simulink model "PubIfDecisionLSM_MDL"  (R2020b)
settings: configuration reference "DspaceConfig" (kept outside this file)
PostLoadFcn:
  | if any(exist('dsrtsu_mdlpostloadfcn', 'file') ~= 0), dsrtsu_mdlpostloadfcn('Execute', bdroot); end
InitFcn:
  | , if any(exist('rtifpga_mdlclblib', 'file') ~= 0), rtifpga_mdlclblib('Init', bdroot); end,
  | , if any(exist('dsmpb_private', 'file') ~= 0), dsmpb_private('dsmpb_mdlclblib', 'Init', bdroot); end,
values from neighbouring files (symbols this model uses):
  P_LSM_ALC_Enable = 0.0    [LSM_Parameter.sldd]
  P_LSM_AwayEdge_offset = 0.1    [LSM_Parameter.sldd]
  P_LSM_CentValidErr = 1.0    [LSM_Parameter.sldd]
  P_LSM_DOP_C0_EN_Limit = 0.8    [LSM_Parameter.sldd]
  P_LSM_DOP_C0_out_Limit = 2.0    [LSM_Parameter.sldd]
  P_LSM_DOP_C1_EN_Limit : value not decoded    [LSM_Parameter.sldd]
  P_LSM_DOP_C1_out_Limit : value not decoded    [LSM_Parameter.sldd]
  P_LSM_DOP_C1AndC2_Lim_X : value not decoded    [LSM_Parameter.sldd]
  P_LSM_DOP_C2_EN_Limit : value not decoded    [LSM_Parameter.sldd]
  P_LSM_DOP_C2_out_Limit : value not decoded    [LSM_Parameter.sldd]
  P_LSM_DOP_In_Pre2Dop_Dis = 1.0    [LSM_Parameter.sldd]
  P_LSM_DOP_Out_Pre2Dop_Dis = 2.0    [LSM_Parameter.sldd]
  P_LSM_DOP_PreDis_X : value not decoded    [LSM_Parameter.sldd]
  P_LSM_DOP_PreDis_Y : value not decoded    [LSM_Parameter.sldd]
  P_LSM_DOPEnableSW = 1.0    [LSM_Parameter.sldd]
  P_LSM_DOPValid_CheckTime = 0.06    [LSM_Parameter.sldd]
  P_LSM_DoubleLine_Curr2Cent_Dislimit = 0.5    [LSM_Parameter.sldd]
  P_LSM_DoubleLine_Dop2Cent_Dislimit = 0.5    [LSM_Parameter.sldd]
  P_LSM_DoubleLine_DOPOut_C1 : value not decoded    [LSM_Parameter.sldd]
  P_LSM_DoubleLine_Pre2Cent_Dislimit = 1.0    [LSM_Parameter.sldd]
  P_LSM_Error_Limit = 0.5    [LSM_Parameter.sldd]
  P_LSM_IFV2CenterAxis = 0.0    [LSM_Parameter.sldd]
  P_LSM_IFV2RearAxis = 0.0    [LSM_Parameter.sldd]
  P_LSM_Line2Edge_limit = 0.5    [LSM_Parameter.sldd]
  P_LSM_Line_Error = 0.1    [LSM_Parameter.sldd]
  P_LSM_LineSTD_Limit = 0.15    [LSM_Parameter.sldd]
  P_LSM_NOH_Switch = 0.0    [LSM_Parameter.sldd]
  P_LSM_OTL_C0_Factor = 1.0    [LSM_Parameter.sldd]
  P_LSM_OTL_C1_Factor = 0.5    [LSM_Parameter.sldd]
  P_LSM_OTL_C2_Factor = 0.5    [LSM_Parameter.sldd]
  P_LSM_Pre2OnlyLineDis = 5.0    [LSM_Parameter.sldd]
  P_LSM_Pre_t = 0.0    [LSM_Parameter.sldd]
  P_LSM_SingleLine_Cent2Edge_Dislimit = 100.0    [LSM_Parameter.sldd]
  P_LSM_SingleLine_Curr2Cent_Dislimit = 0.2    [LSM_Parameter.sldd]
  P_LSM_SingleLine_Dop2Cent_Dislimit = 0.2    [LSM_Parameter.sldd]
  P_LSM_SingleLine_DOPOut_C1 : value not decoded    [LSM_Parameter.sldd]
  P_LSM_SingleLine_Pre2Cent_Dislimit = 0.5    [LSM_Parameter.sldd]
  P_LSM_TJALimitSpd = 60.0    [LSM_Parameter.sldd]
undefined symbols (not defined in the file or in its folder): P_lCS_IFV2CenterAxis, P_LCS_IFV2RearAxis, P_LSM_EntryEdge_offset, P_LSM_EntryLnChngEnSwitch, P_LSM_EntryVanishDis, P_LSM_LinetLostTime, P_LSM_LineWijCal_C12, P_LSM_LineWijCal_C13, P_LSM_MapValid_ErrorSwitch, P_LSM_PosLineLcFac, P_LSM_SpdLim_Stub_Spd, P_LSM_SpdLim_StubLength, P_LSM_SpdTurnAlarm
libraries: simulink x324, TrueDurationTime x11
(part 17 of 25)

== matlab function PubIfDecisionLSM_MDL/Subsystem1/TargetLineCalc_20ms2/LHLine ==
  data: LH_Count input; LH1A0 input single size=1; LH1A1 input single size=1; LH1A2 input single size=1; LH1A3 input single size=1; LH1RaMin input single size=1; LH1RaMax input single size=1; LH1Conf output uint8 size=1; LH1Avail input uint8 size=1; LH1LineType input uint8 size=1; LH1DLType input uint8 size=1; LH1SideType input uint8 size=1; LH1Wid input single size=1; LH1Crossing input; LH1Confidence input; LH1_Color input; LH1DEType input; LH2A0 input single size=1; LH2A1 input single size=1; LH2A2 input single size=1; LH2A3 input single size=1; LH2RaMin input single size=1; LH2RaMax input single size=1; LH2Avail input uint8 size=1; LH2LineType input uint8 size=1; LH2DLType input uint8 size=1; LH2SideType input uint8 size=1; LH2Wid input single size=1; LH1C0 output single size=1; LH1C1 output single size=1; LH1C2 output single size=1; LH1C3 output single size=1; LH1DxMin output single size=1; LH1DxMax output single size=1; LH1Type output uint8 size=1; LH1DLM output uint8 size=1; LH1Width output single size=1; LH1Reliable output; LeftLaneChange output uint8 size=1; LH1Color output; LH1DECEL output; LH2Conf output uint8 size=1; LH2C0 output single size=1; LH2C1 output single size=1; LH2C2 output single size=1; LH2C3 output single size=1; LH2DxMin output single size=1; LH2DxMax output single size=1; LH2Type output uint8 size=1; LH2DLM output uint8 size=1; LH2Width output single size=1; LH2Reliable output; RightLaneChange output uint8 size=1; LH2Crossing input; LH2Confidence input; LH2_Color input; LH2Color output; LH2DEType input; LH2DECEL output
function [LH1Conf,LH1C0,LH1C1,LH1C2,LH1C3,LH1DxMin,LH1DxMax,LH1Type,LH1DLM,LH1Width,LH1Reliable,LeftLaneChange,LH1Color,LH1DECEL,...
    LH2Conf,LH2C0,LH2C1,LH2C2,LH2C3,LH2DxMin,LH2DxMax,LH2Type,LH2DLM,LH2Width,LH2Reliable,RightLaneChange,LH2Color,LH2DECEL]...
    = LH(LH_Count,LH1A0,LH1A1,LH1A2,LH1A3,LH1RaMin,LH1RaMax,LH1Avail,LH1LineType,LH1DLType,LH1SideType,LH1Wid,LH1Crossing,LH1Confidence,LH1_Color,LH1DEType,...
    LH2A0,LH2A1,LH2A2,LH2A3,LH2RaMin,LH2RaMax,LH2Avail,LH2LineType,LH2DLType,LH2SideType,LH2Wid,LH2Crossing,LH2Confidence,LH2_Color,LH2DEType)

LH1Conf = uint8(0);
LH1C0 = single(0);
LH1C1 = single(0);
LH1C2 = single(0);
LH1C3 = single(0);
LH1DxMin = single(0);
LH1DxMax = single(0);
LH1Type = uint8(0);
LH1DLM = uint8(0);
LH1Width = single(0);
LH1Reliable = single(0);
LeftLaneChange = uint8(0);
LH1Color = uint8(0);
LH1DECEL = uint8(0);

LH2Conf = uint8(0);
LH2C0 = single(0);
LH2C1 = single(0);
LH2C2 = single(0);
LH2C3 = single(0);
LH2DxMin = single(0);
LH2DxMax = single(0);
LH2Type = uint8(0);
LH2DLM = uint8(0);
LH2Width = single(0);
LH2Reliable = single(0);
RightLaneChange = uint8(0);
LH2Color = uint8(0);
LH2DECEL = uint8(0);


%%        自车道车道线预处理
if LH_Count >= 1                                       %车道线数量
    if LH1SideType==1                                  %左侧车道线
        LH1Conf = LH1Avail;
        LH1C0 = LH1A0;
        LH1C1 = LH1A1;
        LH1C2 = LH1A2;
        LH1C3 = LH1A3;
        LH1DxMin = LH1RaMin;
        LH1DxMax = LH1RaMax;
        LH1Type = LH1LineType;
        LH1DLM = LH1DLType;
        LH1Width = LH1Wid;
        LH1Reliable = LH1Confidence;
        LeftLaneChange = LH1Crossing;
        LH1Color = LH1_Color;
        LH1DECEL = LH1DEType;
    elseif LH1SideType==2                              %右侧车道线
        LH2Conf = LH1Avail;
        LH2C0 = LH1A0;
        LH2C1 = LH1A1;
        LH2C2 = LH1A2;
        LH2C3 = LH1A3;
        LH2DxMin = LH1RaMin;
        LH2DxMax = LH1RaMax;
        LH2Type = LH1LineType;
        LH2DLM = LH1DLType;
        LH2Width = LH1Wid;
        LH2Reliable = LH1Confidence;
        RightLaneChange = LH1Crossing;
        LH2Color = LH1_Color;
        LH2DECEL = LH1DEType;
    end
    if LH_Count >= 2
        if LH2SideType==1
            LH1Conf = LH2Avail;
            LH1C0 = LH2A0;
            LH1C1 = LH2A1;
            LH1C2 = LH2A2;
            LH1C3 = LH2A3;
            LH1DxMin = LH2RaMin;
            LH1DxMax = LH2RaMax;
            LH1Type = LH2LineType;
            LH1DLM = LH2DLType;
            LH1Width = LH2Wid;
            LH1Reliable = LH2Confidence;
            LeftLaneChange = LH2Crossing;
            LH1Color = LH2_Color;
            LH1DECEL = LH2DEType;
        elseif LH2SideType==2
            LH2Conf = LH2Avail;
            LH2C0 = LH2A0;
            LH2C1 = LH2A1;
            LH2C2 = LH2A2;
            LH2C3 = LH2A3;
            LH2DxMin = LH2RaMin;
            LH2DxMax = LH2RaMax;
            LH2Type = LH2LineType;
            LH2DLM = LH2DLType;
            LH2Width = LH2Wid;
            LH2Reliable = LH2Confidence;
            RightLaneChange = LH2Crossing;
            LH2Color = LH2_Color;
            LH2DECEL = LH2DEType;
        end
    end
end

== matlab function PubIfDecisionLSM_MDL/Subsystem1/TargetLineCalc_20ms2/LHLine1 ==
  data: LHA0 input single size=1; LHA1 input single size=1; LHA2 input single size=1; LHA3 input single size=1; LHRaMin input single size=1; LHRaMax input single size=1; LH_ELEM_Second_C0 input single size=1; LH_ELEM_Second_C1 input single size=1; LH_ELEM_Second_C2 input single size=1; LH_ELEM_Second_C3 input single size=1; LH_ELEM_Second_Start input single size=1; LH_ELEM0_Second_End input single size=1; LHC0 output single size=1; LHC1 output single size=1; LHC2 output single size=1; LHC3 output single size=1; LHDxMin output single size=1; LHDxMax output single size=1; preDis input
function [LHC0,LHC1,LHC2,LHC3,LHDxMin,LHDxMax]...
    = LH(LHA0,LHA1,LHA2,LHA3,LHRaMin,LHRaMax,...
    LH_ELEM_Second_C0,LH_ELEM_Second_C1,LH_ELEM_Second_C2,LH_ELEM_Second_C3,LH_ELEM_Second_Start,LH_ELEM0_Second_End,preDis)

Second_Range = LH_ELEM0_Second_End -LH_ELEM_Second_Start;

if (Second_Range>0.5)&&(preDis>LHRaMax)
    [LineC3,LineC2,LineC1,LineC0,RangeMin,RangeMax]=CurveFitting(LH_ELEM_Second_C0,LH_ELEM_Second_C1,LH_ELEM_Second_C2,LH_ELEM_Second_C3,LH_ELEM_Second_Start,LH_ELEM0_Second_End,...
    LHA0,LHA1,LHA2,LHA3,LHRaMin,LHRaMax,preDis);
            LHC0 = LineC0;
            LHC1 = LineC1;
            LHC2 = LineC2;
            LHC3 = LineC3;
            LHDxMin = RangeMin;
            LHDxMax = RangeMax;
else
    LHC0 = LHA0;
    LHC1 = LHA1;
    LHC2 = LHA2;
    LHC3 = LHA3;
    LHDxMin = LHRaMin;
    LHDxMax = LHRaMax;
end
end

%%


%% 
function [LineC3,LineC2,LineC1,LineC0,RangeMin,RangeMax]=CurveFitting(Second_C0,Second_C1,Second_C2,Second_C3,Second_Start,Second_End,...
    First_C0,First_C1,First_C2,First_C3,First_Start,First_Start_End,preDis)

temp_x = [max(0.2*preDis,First_Start),max(0.6*preDis,First_Start),preDis,1.4*preDis];
if 0.4*preDis<Second_Start
    y1 = First_C0+First_C1*temp_x(1)+First_C2*temp_x(1)^2+First_C3*temp_x(1)^3;
else
    y1 = Second_C0+Second_C1*temp_x(1)+Second_C2*temp_x(1)^2+Second_C3*temp_x(1)^3;
end
if 0.8*preDis<Second_Start
    y2 = First_C0+First_C1*temp_x(2)+First_C2*temp_x(2)^2+First_C3*temp_x(2)^3;
else
    y2 = Second_C0+Second_C1*temp_x(2)+Second_C2*temp_x(2)^2+Second_C3*temp_x(2)^3;
end

if preDis<Second_Start
    y3 = First_C0+First_C1*temp_x(3)+First_C2*temp_x(3)^2+First_C3*temp_x(3)^3;
else
    y3 = Second_C0+Second_C1*temp_x(3)+Second_C2*temp_x(3)^2+Second_C3*temp_x(3)^3;
end

if 1.2*preDis<Second_Start
    y4 = First_C0+First_C1*temp_x(4)+First_C2*temp_x(4)^2+First_C3*temp_x(4)^3;
else
    y4 = Second_C0+Second_C1*temp_x(4)+Second_C2*temp_x(4)^2+Second_C3*temp_x(3)^3;
end
temp_y = [y1,y2,y3,y4];
[LineC3,LineC2,LineC1,LineC0] = pl(temp_x,temp_y);

Range=Second_End-Second_Start;
if Range>0.5
    RangeMin = First_Start;
    RangeMax = 1.2*preDis;
else
    RangeMin = First_Start;
    RangeMax = First_Start_End;
end  
end

== matlab function PubIfDecisionLSM_MDL/Subsystem1/TargetLineCalc_20ms/LHLine ==
  data: LH_Count input; LH1A0 input single size=1; LH1A1 input single size=1; LH1A2 input single size=1; LH1A3 input single size=1; LH1RaMin input single size=1; LH1RaMax input single size=1; LH1Conf output uint8 size=1; LH1Avail input uint8 size=1; LH1LineType input uint8 size=1; LH1DLType input uint8 size=1; LH1SideType input uint8 size=1; LH1Wid input single size=1; LH1Crossing input; LH1Confidence input; LH1_Color input; LH1DEType input; LH2A0 input single size=1; LH2A1 input single size=1; LH2A2 input single size=1; LH2A3 input single size=1; LH2RaMin input single size=1; LH2RaMax input single size=1; LH2Avail input uint8 size=1; LH2LineType input uint8 size=1; LH2DLType input uint8 size=1; LH2SideType input uint8 size=1; LH2Wid input single size=1; LH1C0 output single size=1; LH1C1 output single size=1; LH1C2 output single size=1; LH1C3 output single size=1; LH1DxMin output single size=1; LH1DxMax output single size=1; LH1Type output uint8 size=1; LH1DLM output uint8 size=1; LH1Width output single size=1; LH1Reliable output; LeftLaneChange output uint8 size=1; LH1Color output; LH1DECEL output; LH2Conf output uint8 size=1; LH2C0 output single size=1; LH2C1 output single size=1; LH2C2 output single size=1; LH2C3 output single size=1; LH2DxMin output single size=1; LH2DxMax output single size=1; LH2Type output uint8 size=1; LH2DLM output uint8 size=1; LH2Width output single size=1; LH2Reliable output; RightLaneChange output uint8 size=1; LH2Crossing input; LH2Confidence input; LH2_Color input; LH2Color output; LH2DEType input; LH2DECEL output
function [LH1Conf,LH1C0,LH1C1,LH1C2,LH1C3,LH1DxMin,LH1DxMax,LH1Type,LH1DLM,LH1Width,LH1Reliable,LeftLaneChange,LH1Color,LH1DECEL,...
    LH2Conf,LH2C0,LH2C1,LH2C2,LH2C3,LH2DxMin,LH2DxMax,LH2Type,LH2DLM,LH2Width,LH2Reliable,RightLaneChange,LH2Color,LH2DECEL]...
    = LH(LH_Count,LH1A0,LH1A1,LH1A2,LH1A3,LH1RaMin,LH1RaMax,LH1Avail,LH1LineType,LH1DLType,LH1SideType,LH1Wid,LH1Crossing,LH1Confidence,LH1_Color,LH1DEType,...
    LH2A0,LH2A1,LH2A2,LH2A3,LH2RaMin,LH2RaMax,LH2Avail,LH2LineType,LH2DLType,LH2SideType,LH2Wid,LH2Crossing,LH2Confidence,LH2_Color,LH2DEType)

LH1Conf = uint8(0);
LH1C0 = single(0);
LH1C1 = single(0);
LH1C2 = single(0);
LH1C3 = single(0);
LH1DxMin = single(0);
LH1DxMax = single(0);
LH1Type = uint8(0);
LH1DLM = uint8(0);
LH1Width = single(0);
LH1Reliable = single(0);
LeftLaneChange = uint8(0);
LH1Color = uint8(0);
LH1DECEL = uint8(0);

LH2Conf = uint8(0);
LH2C0 = single(0);
LH2C1 = single(0);
LH2C2 = single(0);
LH2C3 = single(0);
LH2DxMin = single(0);
LH2DxMax = single(0);
LH2Type = uint8(0);
LH2DLM = uint8(0);
LH2Width = single(0);
LH2Reliable = single(0);
RightLaneChange = uint8(0);
LH2Color = uint8(0);
LH2DECEL = uint8(0);


%%        自车道车道线预处理
if LH_Count >= 1                                       %车道线数量
    if LH1SideType==1                                  %左侧车道线
        LH1Conf = LH1Avail;
        LH1C0 = LH1A0;
        LH1C1 = LH1A1;
        LH1C2 = LH1A2;
        LH1C3 = LH1A3;
        LH1DxMin = LH1RaMin;
        LH1DxMax = LH1RaMax;
        LH1Type = LH1LineType;
        LH1DLM = LH1DLType;
        LH1Width = LH1Wid;
        LH1Reliable = LH1Confidence;
        LeftLaneChange = LH1Crossing;
        LH1Color = LH1_Color;
        LH1DECEL = LH1DEType;
    elseif LH1SideType==2                              %右侧车道线
        LH2Conf = LH1Avail;
        LH2C0 = LH1A0;
        LH2C1 = LH1A1;
        LH2C2 = LH1A2;
        LH2C3 = LH1A3;
        LH2DxMin = LH1RaMin;
        LH2DxMax = LH1RaMax;
        LH2Type = LH1LineType;
        LH2DLM = LH1DLType;
        LH2Width = LH1Wid;
        LH2Reliable = LH1Confidence;
        RightLaneChange = LH1Crossing;
        LH2Color = LH1_Color;
        LH2DECEL = LH1DEType;
    end
    if LH_Count >= 2
        if LH2SideType==1
            LH1Conf = LH2Avail;
            LH1C0 = LH2A0;
            LH1C1 = LH2A1;
            LH1C2 = LH2A2;
            LH1C3 = LH2A3;
            LH1DxMin = LH2RaMin;
            LH1DxMax = LH2RaMax;
            LH1Type = LH2LineType;
            LH1DLM = LH2DLType;
            LH1Width = LH2Wid;
            LH1Reliable = LH2Confidence;
            LeftLaneChange = LH2Crossing;
            LH1Color = LH2_Color;
            LH1DECEL = LH2DEType;
        elseif LH2SideType==2
            LH2Conf = LH2Avail;
            LH2C0 = LH2A0;
            LH2C1 = LH2A1;
            LH2C2 = LH2A2;
            LH2C3 = LH2A3;
            LH2DxMin = LH2RaMin;
            LH2DxMax = LH2RaMax;
            LH2Type = LH2LineType;
            LH2DLM = LH2DLType;
            LH2Width = LH2Wid;
            LH2Reliable = LH2Confidence;
            RightLaneChange = LH2Crossing;
            LH2Color = LH2_Color;
            LH2DECEL = LH2DEType;
        end
    end
end

== matlab function PubIfDecisionLSM_MDL/Subsystem1/TargetLineCalc_20ms/LHLine1 ==
  data: LHA0 input single size=1; LHA1 input single size=1; LHA2 input single size=1; LHA3 input single size=1; LHRaMin input single size=1; LHRaMax input single size=1; LH_ELEM_Second_C0 input single size=1; LH_ELEM_Second_C1 input single size=1; LH_ELEM_Second_C2 input single size=1; LH_ELEM_Second_C3 input single size=1; LH_ELEM_Second_Start input single size=1; LH_ELEM_Second_End input single size=1; LHC0 output single size=1; LHC1 output single size=1; LHC2 output single size=1; LHC3 output single size=1; LHDxMin output single size=1; LHDxMax output single size=1
function [LHC0,LHC1,LHC2,LHC3,LHDxMin,LHDxMax]...
    = LH(LHA0,LHA1,LHA2,LHA3,LHRaMin,LHRaMax,...
    LH_ELEM_Second_C0,LH_ELEM_Second_C1,LH_ELEM_Second_C2,LH_ELEM_Second_C3,LH_ELEM_Second_Start,LH_ELEM_Second_End)

Second_Range = LH_ELEM_Second_End -LH_ELEM_Second_Start;

if Second_Range>0.5
%    [LineC3,LineC2,LineC1,LineC0,RangeMin,RangeMax]=CurveFitting(LH_ELEM_Second_C0,LH_ELEM_Second_C1,LH_ELEM_Second_C2,LH_ELEM_Second_C3,LH_ELEM_Second_Start,LH_ELEM0_Second_End,...
%   LHA0,LHA1,LHA2,LHA3,LHRaMin,LHRaMax,preDis);
%             LHC0 = LineC0;
%             LHC1 = LineC1;
%             LHC2 = LineC2;
%             LHC3 = LineC3;
%             LHDxMin = RangeMin;
%             LHDxMax = RangeMax;
    temp_x = [0.3*LHRaMax,0.5*LHRaMax,0.8*LHRaMax,LHRaMax+0.3*(LH_ELEM_Second_End-LH_ELEM_Second_Start),...
        LHRaMax+0.5*(LH_ELEM_Second_End-LH_ELEM_Second_Start),LHRaMax+0.8*(LH_ELEM_Second_End-LH_ELEM_Second_Start)];
  
        y1 = LHA0+LHA1*temp_x(1)+LHA2*temp_x(1)^2+LHA3*temp_x(1)^3;
        y2 = LHA0+LHA1*temp_x(2)+LHA2*temp_x(2)^2+LHA3*temp_x(2)^3;
        y3 = LHA0+LHA1*temp_x(3)+LHA2*temp_x(3)^2+LHA3*temp_x(3)^3;
        y4 = LH_ELEM_Second_C0+LH_ELEM_Second_C1*temp_x(4)+LH_ELEM_Second_C2*temp_x(4)^2+LH_ELEM_Second_C3*temp_x(4)^3;
        y5 = LH_ELEM_Second_C0+LH_ELEM_Second_C1*temp_x(5)+LH_ELEM_Second_C2*temp_x(5)^2+LH_ELEM_Second_C3*temp_x(5)^3;
        y6 = LH_ELEM_Second_C0+LH_ELEM_Second_C1*temp_x(6)+LH_ELEM_Second_C2*temp_x(6)^2+LH_ELEM_Second_C3*temp_x(6)^3;
    temp_y = [y1,y2,y3,y4,y5,y6];
    P = polyfit(temp_x,temp_y,2);
    LHC3 = single(0);
    LHC2 = P(1);
    LHC1 = P(2);
    LHC0 = P(3);
    Range=LH_ELEM_Second_End-LH_ELEM_Second_Start;
    if Range>0.5
        LHDxMin = LHRaMin;
        LHDxMax = LH_ELEM_Second_End;
    else
         LHDxMin = LHRaMin;
         LHDxMax = LHRaMax;
    end
else
    LHC0 = LHA0;
    LHC1 = LHA1;
    LHC2 = LHA2;
    LHC3 = LHA3;
    LHDxMin = LHRaMin;
    LHDxMax = LHRaMax;
end
end

%%


%% 
% function [LineC3,LineC2,LineC1,LineC0,RangeMin,RangeMax]=CurveFitting(Second_C0,Second_C1,Second_C2,Second_C3,Second_Start,Second_End,...
%     First_C0,First_C1,First_C2,First_C3,First_Start,First_Start_End,preDis)
% 
% temp_x = [0.4*preDis,0.8*preDis,preDis,1.2*preDis];
% if 0.4*preDis<Second_Start
%     y1 = First_C0+First_C1*temp_x(1)+First_C2*temp_x(1)^2+First_C3*temp_x(1)^3;
% else
%     y1 = Second_C0+Second_C1*temp_x(1)+Second_C2*temp_x(1)^2+Second_C3*temp_x(1)^3;
% end
% if 0.8*preDis<Second_Start
%     y2 = First_C0+First_C1*temp_x(2)+First_C2*temp_x(2)^2+First_C3*temp_x(2)^3;
% else
%     y2 = Second_C0+Second_C1*temp_x(2)+Second_C2*temp_x(2)^2+Second_C3*temp_x(2)^3;
% end
% 
% if preDis<Second_Start
%     y3 = First_C0+First_C1*temp_x(3)+First_C2*temp_x(3)^2+First_C3*temp_x(3)^3;
% else
%     y3 = Second_C0+Second_C1*temp_x(3)+Second_C2*temp_x(3)^2+Second_C3*temp_x(3)^3;
% end
% 
% if 1.2*preDis<Second_Start
%     y4 = First_C0+First_C1*temp_x(4)+First_C2*temp_x(4)^2+First_C3*temp_x(4)^3;
% else
%     y4 = Second_C0+Second_C1*temp_x(4)+Second_C2*temp_x(4)^2+Second_C3*temp_x(3)^3;
% end
% temp_y = [y1,y2,y3,y4];
% [LineC3,LineC2,LineC1,LineC0] = pl(temp_x,temp_y);
% 
% Range=Second_End-Second_Start;
% if Range>0.5
%     RangeMin = First_Start;
%     RangeMax = Second_End;
% else
%     RangeMin = First_Start;
%     RangeMax = First_Start_End;
% end  
% end

== matlab function PubIfDecisionLSM_MDL/Subsystem1/TargetLineCalc_20ms/LHLine2 ==
  data: LHA0 input single size=1; LHA1 input single size=1; LHA2 input single size=1; LHA3 input single size=1; LHRaMin input single size=1; LHRaMax input single size=1; LH_ELEM_Second_C0 input single size=1; LH_ELEM_Second_C1 input single size=1; LH_ELEM_Second_C2 input single size=1; LH_ELEM_Second_C3 input single size=1; LH_ELEM_Second_Start input single size=1; LH_ELEM_Second_End input single size=1; LHC0 output single size=1; LHC1 output single size=1; LHC2 output single size=1; LHC3 output single size=1; LHDxMin output single size=1; LHDxMax output single size=1
function [LHC0,LHC1,LHC2,LHC3,LHDxMin,LHDxMax]...
    = LH(LHA0,LHA1,LHA2,LHA3,LHRaMin,LHRaMax,...
    LH_ELEM_Second_C0,LH_ELEM_Second_C1,LH_ELEM_Second_C2,LH_ELEM_Second_C3,LH_ELEM_Second_Start,LH_ELEM_Second_End)

Second_Range = LH_ELEM_Second_End -LH_ELEM_Second_Start;

if Second_Range>0.5
%    [LineC3,LineC2,LineC1,LineC0,RangeMin,RangeMax]=CurveFitting(LH_ELEM_Second_C0,LH_ELEM_Second_C1,LH_ELEM_Second_C2,LH_ELEM_Second_C3,LH_ELEM_Second_Start,LH_ELEM0_Second_End,...
%   LHA0,LHA1,LHA2,LHA3,LHRaMin,LHRaMax,preDis);
%             LHC0 = LineC0;
%             LHC1 = LineC1;
%             LHC2 = LineC2;
%             LHC3 = LineC3;
%             LHDxMin = RangeMin;
%             LHDxMax = RangeMax;
    temp_x = [0.3*LHRaMax,0.5*LHRaMax,0.8*LHRaMax,LHRaMax+0.3*(LH_ELEM_Second_End-LH_ELEM_Second_Start),...
        LHRaMax+0.5*(LH_ELEM_Second_End-LH_ELEM_Second_Start),LHRaMax+0.8*(LH_ELEM_Second_End-LH_ELEM_Second_Start)];
  
        y1 = LHA0+LHA1*temp_x(1)+LHA2*temp_x(1)^2+LHA3*temp_x(1)^3;
        y2 = LHA0+LHA1*temp_x(2)+LHA2*temp_x(2)^2+LHA3*temp_x(2)^3;
        y3 = LHA0+LHA1*temp_x(3)+LHA2*temp_x(3)^2+LHA3*temp_x(3)^3;
        y4 = LH_ELEM_Second_C0+LH_ELEM_Second_C1*temp_x(4)+LH_ELEM_Second_C2*temp_x(4)^2+LH_ELEM_Second_C3*temp_x(4)^3;
        y5 = LH_ELEM_Second_C0+LH_ELEM_Second_C1*temp_x(5)+LH_ELEM_Second_C2*temp_x(5)^2+LH_ELEM_Second_C3*temp_x(5)^3;
        y6 = LH_ELEM_Second_C0+LH_ELEM_Second_C1*temp_x(6)+LH_ELEM_Second_C2*temp_x(6)^2+LH_ELEM_Second_C3*temp_x(6)^3;
    temp_y = [y1,y2,y3,y4,y5,y6];
    P = polyfit(temp_x,temp_y,2);
    LHC3 = single(0);
    LHC2 = P(1);
    LHC1 = P(2);
    LHC0 = P(3);
    Range=LH_ELEM_Second_End-LH_ELEM_Second_Start;
    if Range>0.5
        LHDxMin = LHRaMin;
        LHDxMax = LH_ELEM_Second_End;
    else
         LHDxMin = LHRaMin;
         LHDxMax = LHRaMax;
    end
else
    LHC0 = LHA0;
    LHC1 = LHA1;
    LHC2 = LHA2;
    LHC3 = LHA3;
    LHDxMin = LHRaMin;
    LHDxMax = LHRaMax;
end
end

%%


%% 
% function [LineC3,LineC2,LineC1,LineC0,RangeMin,RangeMax]=CurveFitting(Second_C0,Second_C1,Second_C2,Second_C3,Second_Start,Second_End,...
%     First_C0,First_C1,First_C2,First_C3,First_Start,First_Start_End,preDis)
% 
% temp_x = [0.4*preDis,0.8*preDis,preDis,1.2*preDis];
% if 0.4*preDis<Second_Start
%     y1 = First_C0+First_C1*temp_x(1)+First_C2*temp_x(1)^2+First_C3*temp_x(1)^3;
% else
%     y1 = Second_C0+Second_C1*temp_x(1)+Second_C2*temp_x(1)^2+Second_C3*temp_x(1)^3;
% end
% if 0.8*preDis<Second_Start
%     y2 = First_C0+First_C1*temp_x(2)+First_C2*temp_x(2)^2+First_C3*temp_x(2)^3;
% else
%     y2 = Second_C0+Second_C1*temp_x(2)+Second_C2*temp_x(2)^2+Second_C3*temp_x(2)^3;
% end
% 
% if preDis<Second_Start
%     y3 = First_C0+First_C1*temp_x(3)+First_C2*temp_x(3)^2+First_C3*temp_x(3)^3;
% else
%     y3 = Second_C0+Second_C1*temp_x(3)+Second_C2*temp_x(3)^2+Second_C3*temp_x(3)^3;
% end
% 
% if 1.2*preDis<Second_Start
%     y4 = First_C0+First_C1*temp_x(4)+First_C2*temp_x(4)^2+First_C3*temp_x(4)^3;
% else
%     y4 = Second_C0+Second_C1*temp_x(4)+Second_C2*temp_x(4)^2+Second_C3*temp_x(3)^3;
% end
% temp_y = [y1,y2,y3,y4];
% [LineC3,LineC2,LineC1,LineC0] = pl(temp_x,temp_y);
% 
% Range=Second_End-Second_Start;
% if Range>0.5
%     RangeMin = First_Start;
%     RangeMax = Second_End;
% else
%     RangeMin = First_Start;
%     RangeMax = First_Start_End;
% end  
% end

== matlab function PubIfDecisionLSM_MDL/Subsystem1/TargetLineCalc_20ms/LRELine ==
  data: LRE_Count input uint8 size=1; LRE1A0 input single size=1; LRE1A1 input single size=1; LRE1A2 input single size=1; LRE1A3 input single size=1; LRE1RaMin input single size=1; LRE1RaMax input single size=1; LRE1Conf output uint8 size=1; LRE1Avail input uint8 size=1; LRE1SideType input uint8 size=1; LRE1Confdience input; LRE2A0 input single size=1; LRE2A1 input single size=1; LRE2A2 input single size=1; LRE2A3 input single size=1; LRE2RaMin input single size=1; LRE2RaMax input single size=1; LRE2Avail input uint8 size=1; LRE2SideType input uint8 size=1; LRE1C0 output single size=1; LRE1C1 output single size=1; LRE1C2 output single size=1; LRE1C3 output single size=1; LRE1DxMin output single size=1; LRE1DxMax output single size=1; LRE1Reliable output; LRE2Conf output uint8 size=1; LRE2C0 output single size=1; LRE2C1 output single size=1; LRE2C2 output single size=1; LRE2C3 output single size=1; LRE2DxMin output single size=1; LRE2DxMax output single size=1; LRE2Confdience input; LRE2Reliable output
function [LRE1Conf,LRE1C0,LRE1C1,LRE1C2,LRE1C3,LRE1DxMin,LRE1DxMax,LRE1Reliable,...
    LRE2Conf,LRE2C0,LRE2C1,LRE2C2,LRE2C3,LRE2DxMin,LRE2DxMax,LRE2Reliable]...
    = LRE(LRE_Count,LRE1A0,LRE1A1,LRE1A2,LRE1A3,LRE1RaMin,LRE1RaMax,LRE1Avail,LRE1SideType,LRE1Confdience,...
    LRE2A0,LRE2A1,LRE2A2,LRE2A3,LRE2RaMin,LRE2RaMax,LRE2Avail,LRE2SideType,LRE2Confdience)

LRE1Conf = uint8(0);
LRE1C0 = single(0);
LRE1C1 = single(0);
LRE1C2 = single(0);
LRE1C3 = single(0);
LRE1DxMin = single(0);
LRE1DxMax = single(0);
LRE1Reliable = single(0);

LRE2Conf = uint8(0);
LRE2C0 = single(0);
LRE2C1 = single(0);
LRE2C2 = single(0);
LRE2C3 = single(0);
LRE2DxMin = single(0);
LRE2DxMax = single(0);
LRE2Reliable = single(0);

%%     边界线预处理
if LRE_Count == 2                                   %边界线数量
    if LRE1SideType==1                              %左侧边界线
        LRE1Conf = LRE1Avail;
        LRE1C0 = LRE1A0;
        LRE1C1 = LRE1A1;
        LRE1C2 = LRE1A2;
        LRE1C3 = LRE1A3;
        LRE1DxMin = LRE1RaMin;
        LRE1DxMax = LRE1RaMax;
        LRE1Reliable = LRE1Confdience;
    elseif LRE1SideType==2                           %右侧边界线
        LRE2Conf = LRE1Avail;
        LRE2C0 = LRE1A0;
        LRE2C1 = LRE1A1;
        LRE2C2 = LRE1A2;
        LRE2C3 = LRE1A3;
        LRE2DxMin = LRE1RaMin;
        LRE2DxMax = LRE1RaMax;
        LRE2Reliable = LRE1Confdience;
    end
    
    if LRE2SideType==1
        LRE1Conf = LRE2Avail;
        LRE1C0 = LRE2A0;
        LRE1C1 = LRE2A1;
        LRE1C2 = LRE2A2;
        LRE1C3 = LRE2A3;
        LRE1DxMin = LRE2RaMin;
        LRE1DxMax = LRE2RaMax;
        LRE1Reliable = LRE2Confdience;
    elseif LRE2SideType==2
        LRE2Conf = LRE2Avail;
        LRE2C0 = LRE2A0;
        LRE2C1 = LRE2A1;
        LRE2C2 = LRE2A2;
        LRE2C3 = LRE2A3;
        LRE2DxMin = LRE2RaMin;
        LRE2DxMax = LRE2RaMax;
        LRE2Reliable = LRE2Confdience;
    end
end

%%
if LRE_Count == 1
    if LRE1SideType==1
        LRE1Conf = LRE1Avail;
        LRE1C0 = LRE1A0;
        LRE1C1 = LRE1A1;
        LRE1C2 = LRE1A2;
        LRE1C3 = LRE1A3;
        LRE1DxMin = LRE1RaMin;
        LRE1DxMax = LRE1RaMax;
        LRE1Reliable = LRE1Confdience;
    elseif LRE1SideType==2
        LRE2Conf = LRE1Avail;
        LRE2C0 = LRE1A0;
        LRE2C1 = LRE1A1;
        LRE2C2 = LRE1A2;
        LRE2C3 = LRE1A3;
        LRE2DxMin = LRE1RaMin;
        LRE2DxMax = LRE1RaMax;
        LRE2Reliable = LRE1Confdience;
    end
end

== matlab function PubIfDecisionLSM_MDL/Subsystem1/TargetLineCalc_20ms/MATLAB Function ==
  data: LA_Sync_ID input uint8 size=1; y output boolean size=1; LA_Update input boolean size=1; LH_Sync_ID input uint8 size=1; LH_Upadate input boolean size=1
function y = fcn(LA_Sync_ID,LA_Update,LH_Sync_ID,LH_Upadate)
if (LA_Sync_ID==LH_Sync_ID) && (LA_Update==true||LH_Upadate==true)
    y = true;
else
    y = false;
end

== matlab function PubIfDecisionLSM_MDL/Subsystem1/TargetLineCalc_20ms/TargetLineCalc/Subsystem5/MATLAB Function6 ==
  data: kap input; preDis input; CentLineValidK1 input; CentLineC3K1 input; CentLineC2K1 input; CentLineC1K1 input; CentLineC0K1 input; VisLineA3 input; VisLineA2 input; VisLineA1 input; VisLineA0 input; n1 input; n2 input; CosOfPsi input; SinOfPsi input; dDeltaX input; dDeltaY input; d_cur2 output; delta_d2 output; d_cur3 output; delta_d3 output; HWASts input
function [d_cur2,delta_d2,d_cur3,delta_d3] = ...
    fcn( kap,preDis,CentLineValidK1,CentLineC3K1,CentLineC2K1,CentLineC1K1,CentLineC0K1,...
    VisLineA3,VisLineA2,VisLineA1,VisLineA0,n1,n2,...
    CosOfPsi,SinOfPsi,dDeltaX,dDeltaY, HWASts)

xi = [single(1);single(2);single(3);single(4)];
yi = CentLineC3K1*xi.^3 + CentLineC2K1*xi.^2 + CentLineC1K1*xi + CentLineC0K1;
t_dx = xi-dDeltaX;
t_dy = yi-dDeltaY;
TmpX = t_dx*CosOfPsi+t_dy*SinOfPsi;
TmpY = -t_dx*SinOfPsi+t_dy*CosOfPsi;
[t3,t2,t1,t0] = pl(TmpX,TmpY);

if CentLineValidK1
    m1 = n1;
    m2 = n2;
else
    m1 = single(0);
    m2 = single(0);
end


RefA3_2 = t3*m1;
RefA2_2 = t2*m1 + (1-m1)*(0.5*kap);
RefA1_2 = t1*m1;
RefA0_2 = t0*m1;

RefA3_3 = t3*m2;
RefA2_3 = t2*m2 + (1-m2)*(0.5*kap);
RefA1_3 = t1*m2;
RefA0_3 = t0*m2;

y2 = RefA3_2*(preDis^3) + RefA2_2*(preDis^2) + RefA1_2*preDis + RefA0_2;
y3 = RefA3_3*(preDis^3) + RefA2_3*(preDis^2) + RefA1_3*preDis + RefA0_3;

if HWASts == 5 ||HWASts == 6
    d_cur2 = abs( VisLineA0(2) - RefA0_2);
    d_cur3 = abs(RefA0_3 - VisLineA0(3));
else
    d_cur2 = VisLineA0(2) - RefA0_2;
    d_cur3 = RefA0_3 - VisLineA0(3);
end


d_pre2 = abs((VisLineA0(2) + VisLineA1(2)*preDis + VisLineA2(2)*(preDis^2) + VisLineA3(2)*(preDis^3)) - y2);  %预瞄点的距离
d_pre3 = abs((VisLineA0(3) + VisLineA1(3)*preDis + VisLineA2(3)*(preDis^2) + VisLineA3(3)*(preDis^3)) - y3);
delta_d2 = abs(d_pre2 - d_cur2);
delta_d3 = abs(d_pre3 - d_cur3);

== matlab function PubIfDecisionLSM_MDL/Subsystem1/TargetLineCalc_20ms/TargetLineCalc/Subsystem5/MATLAB Function7 ==
  data: dy2_Ran output; L2_R input; dy3_Ran output; L3_R input
function [dy2_Ran,dy3_Ran] = fcn(L2_R,L3_R)
dy2_Ran = L2_R;
dy3_Ran= L3_R;

== matlab function PubIfDecisionLSM_MDL/Subsystem1/TargetLineCalc_20ms/TargetLineCalc/Subsystem5/MATLAB Function8 ==
  data: VisLineReliable input; dy2_Rel output; dy3_Rel output
function [dy2_Rel,dy3_Rel] = fcn(VisLineReliable)
dy2_Rel = VisLineReliable(2);
dy3_Rel = VisLineReliable(3);

== matlab function PubIfDecisionLSM_MDL/Subsystem1/TargetLineCalc_20ms2/LHLine2 ==
  data: LHA0 input single size=1; LHA1 input single size=1; LHA2 input single size=1; LHA3 input single size=1; LHRaMin input single size=1; LHRaMax input single size=1; LH_ELEM_Second_C0 input single size=1; LH_ELEM_Second_C1 input single size=1; LH_ELEM_Second_C2 input single size=1; LH_ELEM_Second_C3 input single size=1; LH_ELEM_Second_Start input single size=1; LH_ELEM0_Second_End input single size=1; LHC0 output single size=1; LHC1 output single size=1; LHC2 output single size=1; LHC3 output single size=1; LHDxMin output single size=1; LHDxMax output single size=1; preDis input
function [LHC0,LHC1,LHC2,LHC3,LHDxMin,LHDxMax]...
    = LH(LHA0,LHA1,LHA2,LHA3,LHRaMin,LHRaMax,...
    LH_ELEM_Second_C0,LH_ELEM_Second_C1,LH_ELEM_Second_C2,LH_ELEM_Second_C3,LH_ELEM_Second_Start,LH_ELEM0_Second_End,preDis)

Second_Range = LH_ELEM0_Second_End -LH_ELEM_Second_Start;

if (Second_Range>0.5)&&(preDis>LHRaMax)
    [LineC3,LineC2,LineC1,LineC0,RangeMin,RangeMax]=CurveFitting(LH_ELEM_Second_C0,LH_ELEM_Second_C1,LH_ELEM_Second_C2,LH_ELEM_Second_C3,LH_ELEM_Second_Start,LH_ELEM0_Second_End,...
    LHA0,LHA1,LHA2,LHA3,LHRaMin,LHRaMax,preDis);
            LHC0 = LineC0;
            LHC1 = LineC1;
            LHC2 = LineC2;
            LHC3 = LineC3;
            LHDxMin = RangeMin;
            LHDxMax = RangeMax;
else
    LHC0 = LHA0;
    LHC1 = LHA1;
    LHC2 = LHA2;
    LHC3 = LHA3;
    LHDxMin = LHRaMin;
    LHDxMax = LHRaMax;
end
end

%%


%% 
function [LineC3,LineC2,LineC1,LineC0,RangeMin,RangeMax]=CurveFitting(Second_C0,Second_C1,Second_C2,Second_C3,Second_Start,Second_End,...
    First_C0,First_C1,First_C2,First_C3,First_Start,First_Start_End,preDis)

temp_x = [max(0.4*preDis,First_Start),max(0.8*preDis,First_Start),preDis,1.4*preDis];
if 0.4*preDis<Second_Start
    y1 = First_C0+First_C1*temp_x(1)+First_C2*temp_x(1)^2+First_C3*temp_x(1)^3;
else
    y1 = Second_C0+Second_C1*temp_x(1)+Second_C2*temp_x(1)^2+Second_C3*temp_x(1)^3;
end
if 0.8*preDis<Second_Start
    y2 = First_C0+First_C1*temp_x(2)+First_C2*temp_x(2)^2+First_C3*temp_x(2)^3;
else
    y2 = Second_C0+Second_C1*temp_x(2)+Second_C2*temp_x(2)^2+Second_C3*temp_x(2)^3;
end

if preDis<Second_Start
    y3 = First_C0+First_C1*temp_x(3)+First_C2*temp_x(3)^2+First_C3*temp_x(3)^3;
else
    y3 = Second_C0+Second_C1*temp_x(3)+Second_C2*temp_x(3)^2+Second_C3*temp_x(3)^3;
end

if 1.2*preDis<Second_Start
    y4 = First_C0+First_C1*temp_x(4)+First_C2*temp_x(4)^2+First_C3*temp_x(4)^3;
else
    y4 = Second_C0+Second_C1*temp_x(4)+Second_C2*temp_x(4)^2+Second_C3*temp_x(3)^3;
end
temp_y = [y1,y2,y3,y4];
[LineC3,LineC2,LineC1,LineC0] = pl(temp_x,temp_y);

Range=Second_End-Second_Start;
if Range>0.5
    RangeMin = max(0.4*preDis,First_Start);
    RangeMax = 1.2*preDis;
else
    RangeMin = First_Start;
    RangeMax = First_Start_End;
end  
end

== matlab function PubIfDecisionLSM_MDL/Subsystem1/TargetLineCalc_20ms2/LRELine ==
  data: LRE_Count input uint8 size=1; LRE1A0 input single size=1; LRE1A1 input single size=1; LRE1A2 input single size=1; LRE1A3 input single size=1; LRE1RaMin input single size=1; LRE1RaMax input single size=1; LRE1Conf output uint8 size=1; LRE1Avail input uint8 size=1; LRE1SideType input uint8 size=1; LRE1Confdience input; LRE2A0 input single size=1; LRE2A1 input single size=1; LRE2A2 input single size=1; LRE2A3 input single size=1; LRE2RaMin input single size=1; LRE2RaMax input single size=1; LRE2Avail input uint8 size=1; LRE2SideType input uint8 size=1; LRE1C0 output single size=1; LRE1C1 output single size=1; LRE1C2 output single size=1; LRE1C3 output single size=1; LRE1DxMin output single size=1; LRE1DxMax output single size=1; LRE1Reliable output; LRE2Conf output uint8 size=1; LRE2C0 output single size=1; LRE2C1 output single size=1; LRE2C2 output single size=1; LRE2C3 output single size=1; LRE2DxMin output single size=1; LRE2DxMax output single size=1; LRE2Confdience input; LRE2Reliable output
function [LRE1Conf,LRE1C0,LRE1C1,LRE1C2,LRE1C3,LRE1DxMin,LRE1DxMax,LRE1Reliable,...
    LRE2Conf,LRE2C0,LRE2C1,LRE2C2,LRE2C3,LRE2DxMin,LRE2DxMax,LRE2Reliable]...
    = LRE(LRE_Count,LRE1A0,LRE1A1,LRE1A2,LRE1A3,LRE1RaMin,LRE1RaMax,LRE1Avail,LRE1SideType,LRE1Confdience,...
    LRE2A0,LRE2A1,LRE2A2,LRE2A3,LRE2RaMin,LRE2RaMax,LRE2Avail,LRE2SideType,LRE2Confdience)

LRE1Conf = uint8(0);
LRE1C0 = single(0);
LRE1C1 = single(0);
LRE1C2 = single(0);
LRE1C3 = single(0);
LRE1DxMin = single(0);
LRE1DxMax = single(0);
LRE1Reliable = single(0);

LRE2Conf = uint8(0);
LRE2C0 = single(0);
LRE2C1 = single(0);
LRE2C2 = single(0);
LRE2C3 = single(0);
LRE2DxMin = single(0);
LRE2DxMax = single(0);
LRE2Reliable = single(0);

%%     边界线预处理
if LRE_Count == 2                                   %边界线数量
    if LRE1SideType==1                              %左侧边界线
        LRE1Conf = LRE1Avail;
        LRE1C0 = LRE1A0;
        LRE1C1 = LRE1A1;
        LRE1C2 = LRE1A2;
        LRE1C3 = LRE1A3;
        LRE1DxMin = LRE1RaMin;
        LRE1DxMax = LRE1RaMax;
        LRE1Reliable = LRE1Confdience;
    elseif LRE1SideType==2                           %右侧边界线
        LRE2Conf = LRE1Avail;
        LRE2C0 = LRE1A0;
        LRE2C1 = LRE1A1;
        LRE2C2 = LRE1A2;
        LRE2C3 = LRE1A3;
        LRE2DxMin = LRE1RaMin;
        LRE2DxMax = LRE1RaMax;
        LRE2Reliable = LRE1Confdience;
    end
    
    if LRE2SideType==1
        LRE1Conf = LRE2Avail;
        LRE1C0 = LRE2A0;
        LRE1C1 = LRE2A1;
        LRE1C2 = LRE2A2;
        LRE1C3 = LRE2A3;
        LRE1DxMin = LRE2RaMin;
        LRE1DxMax = LRE2RaMax;
        LRE1Reliable = LRE2Confdience;
    elseif LRE2SideType==2
        LRE2Conf = LRE2Avail;
        LRE2C0 = LRE2A0;
        LRE2C1 = LRE2A1;
        LRE2C2 = LRE2A2;
        LRE2C3 = LRE2A3;
        LRE2DxMin = LRE2RaMin;
        LRE2DxMax = LRE2RaMax;
        LRE2Reliable = LRE2Confdience;
    end
end

%%
if LRE_Count == 1
    if LRE1SideType==1
        LRE1Conf = LRE1Avail;
        LRE1C0 = LRE1A0;
        LRE1C1 = LRE1A1;
        LRE1C2 = LRE1A2;
        LRE1C3 = LRE1A3;
        LRE1DxMin = LRE1RaMin;
        LRE1DxMax = LRE1RaMax;
        LRE1Reliable = LRE1Confdience;
    elseif LRE1SideType==2
        LRE2Conf = LRE1Avail;
        LRE2C0 = LRE1A0;
        LRE2C1 = LRE1A1;
        LRE2C2 = LRE1A2;
        LRE2C3 = LRE1A3;
        LRE2DxMin = LRE1RaMin;
        LRE2DxMax = LRE1RaMax;
        LRE2Reliable = LRE1Confdience;
    end
end

== matlab function PubIfDecisionLSM_MDL/Subsystem1/TargetLineCalc_20ms2/MATLAB Function ==
  data: LA_Sync_ID input uint8 size=1; y output boolean size=1; LA_Update input boolean size=1; LH_Sync_ID input uint8 size=1; LH_Upadate input boolean size=1
function y = fcn(LA_Sync_ID,LA_Update,LH_Sync_ID,LH_Upadate)
if (LA_Sync_ID==LH_Sync_ID) && (LA_Update==true||LH_Upadate==true)
    y = true;
else
    y = false;
end

== matlab function PubIfDecisionLSM_MDL/Subsystem1/TargetLineCalc_20ms2/Simulink Function/MATLAB Function3 ==
  data: IFV2RearAxis input single size=1; a0 output single size=1; a1 output single size=1; a2 output single size=1; a3 output single size=1; IFV2CenterAxis input single size=1; A0 input single size=1; A1 input single size=1; A2 input single size=1; A3 input single size=1; Range_min input single size=1; Rmin output single size=1; Range_max input single size=1; Rmax output single size=1
function [a0,a1,a2,a3,Rmin,Rmax] = ...
    fcn(IFV2RearAxis,IFV2CenterAxis,A0,A1,A2,A3,Range_min,Range_max)

Rmin = Range_min + IFV2RearAxis;
Rmax = Range_max + IFV2RearAxis;

if Range_max>0
   xi = [10;20;40;80];
   yi = -A3*xi.^3 - A2*xi.^2 - A1*xi - A0 + IFV2CenterAxis;
   xi = xi + IFV2RearAxis;
   [a3,a2,a1,a0] = pl(xi,yi);
else
    a3 = single(0);
    a2 = single(0);
    a1 = single(0);
    a0 = single(0);
end

== matlab function PubIfDecisionLSM_MDL/Subsystem1/TargetLineCalc_20ms2/TargetLineCalc/CalcEgoVehMove ==
  data: dDeltaX output single size=1; tCycle input single size=1; Kap input single size=1; Vego input single size=1; dDeltaY output single size=1; CosOfPsi output single size=1; SinOfPsi output single size=1
function [dDeltaX,dDeltaY,CosOfPsi,SinOfPsi] = EgoVehicleMovement(tCycle,Kap,Vego)
%#codegen
if Kap==0
    dDeltaX = Vego*tCycle;
    dDeltaY = single(0);
    CosOfPsi = single(1);
    SinOfPsi = single(0);
else
    t_Psi = Kap*Vego*tCycle;
    SinOfPsi = sin(t_Psi);
    CosOfPsi = cos(t_Psi);
    dDeltaX = SinOfPsi/Kap;
    dDeltaY = 2*(sin(t_Psi/2)*sin(t_Psi/2))/Kap;
end

== matlab function PubIfDecisionLSM_MDL/Subsystem1/TargetLineCalc_20ms2/TargetLineCalc/CalcEgoVehMove1 ==
  data: dDeltaX output single size=1; tCycle input single size=1; Kap input single size=1; Vego input single size=1; dDeltaY output single size=1; CosOfPsi output single size=1; SinOfPsi output single size=1
function [dDeltaX,dDeltaY,CosOfPsi,SinOfPsi] = EgoVehicleMovement(tCycle,Kap,Vego)
%#codegen
if Kap==0
    dDeltaX = Vego*tCycle;
    dDeltaY = single(0);
    CosOfPsi = single(1);
    SinOfPsi = single(0);
else
    t_Psi = Kap*Vego*tCycle;
    SinOfPsi = sin(t_Psi);
    CosOfPsi = cos(t_Psi);
    dDeltaX = SinOfPsi/Kap;
    dDeltaY = 2*(sin(t_Psi/2)*sin(t_Psi/2))/Kap;
end

== matlab function PubIfDecisionLSM_MDL/Subsystem1/TargetLineCalc_20ms2/TargetLineCalc/CalcEgoVehMove2 ==
  data: dDeltaX output single size=1; tCycle input single size=1; Kap input single size=1; Vego input single size=1; dDeltaY output single size=1; CosOfPsi output single size=1; SinOfPsi output single size=1
function [dDeltaX,dDeltaY,CosOfPsi,SinOfPsi] = EgoVehicleMovement(tCycle,Kap,Vego)
%#codegen
if Kap==0
    dDeltaX = Vego*tCycle;
    dDeltaY = single(0);
    CosOfPsi = single(1);
    SinOfPsi = single(0);
else
    t_Psi = Kap*Vego*tCycle;
    SinOfPsi = sin(t_Psi);
    CosOfPsi = cos(t_Psi);
    dDeltaX = SinOfPsi/Kap;
    dDeltaY = 2*(sin(t_Psi/2)*sin(t_Psi/2))/Kap;
end
